simulink model "loberotator_final"  (R2018a)
settings: Solver=VariableStepAuto  StartTime=0.0  StopTime=100  RelTol=1e-3
libraries: xbsIndex_r4 x104, xps_library x4, casper_library_misc x1
(part 3 of 4)

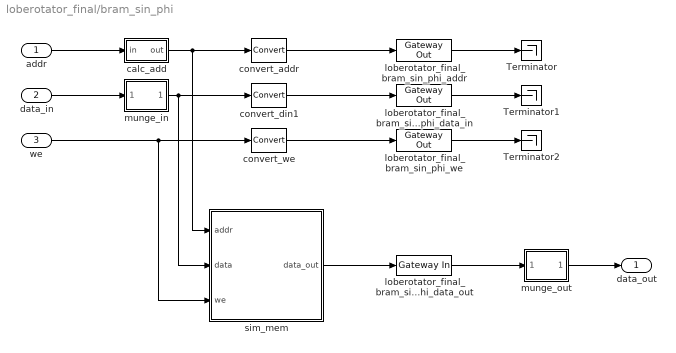
== system loberotator_final/bram_sin_phi ==
  addr : Inport
  data_in : Inport  Port=2
  we : Inport  Port=3
  Terminator : Terminator
  Terminator1 : Terminator
  Terminator2 : Terminator
  calc_add : Subsystem  mask{data_width=32, addr_width=11, sample_rate=sample_rate}
      mask prompts: data_width "data width"; addr_width "address width"; sample_rate "sample rate"
  convert_addr : xbsIndex_r4/Convert  gui_display_data_type=Fixed-point  arith_type=Unsigned  n_bits=addr_width  bin_pt=0  float_type=Single  exp_bits=8  fraction_bits=24  quantization=Truncate  overflow=Wrap  en=off  latency=0  pipeline=off  dbl_ovrd=off  block_type=convert
      settings: xl_area=[0, 0, 0, 0, 0, 0, 0]
  convert_din1 : xbsIndex_r4/Convert  gui_display_data_type=Fixed-point  arith_type=Unsigned  n_bits=32  bin_pt=0  float_type=Single  exp_bits=8  fraction_bits=24  quantization=Truncate  overflow=Wrap  en=off  latency=0  pipeline=off  dbl_ovrd=off  block_type=convert
      settings: xl_area=[0, 0, 0, 0, 0, 0, 0]
  convert_we : xbsIndex_r4/Convert  gui_display_data_type=Fixed-point  arith_type=Unsigned  n_bits=1  bin_pt=0  float_type=Single  exp_bits=8  fraction_bits=24  quantization=Truncate  overflow=Wrap  en=off  latency=0  pipeline=off  dbl_ovrd=off  block_type=convert
      settings: xl_area=[0, 0, 0, 0, 0, 0, 0]
  loberotator_final_bram_sin_phi_addr : xbsIndex_r4/Gateway Out  inherit_from_input=off  hdl_port=on  rows=1  columns=1  UseAsDAC=off  DACChannel='1'  interface=None  automatic_assignment=on  address_offset=hex2dec('00')  intf_name=''  intf_description=''  timing_constraint=None  locs_specified=off  LOCs={'A5','B9','A9','C1','A3','G6','E9','A6','A7','A8','B8','B1','B3','D9','B5','B4','B6','C2'}  io_standard={}  block_type=gatewayout
      settings: infoedit="Gateway out block.  Converts Xilinx fixed point inputs into ouputs of type Simulink integer, double, or fixed point.<P><P>Hardware notes:  In hardware these blocks become top level output ports or are discarded, depending on how they are configured."  sginterface={'Nallatech'=>{'xdspkit'=>{'non_memory_mapped_port'=>'uprev_Shared_BRAM_addr'}},'Xilinx'=>{'jtaghwcosim'=>{'non_memory_mapped_port'=>'uprev_Shared_BRAM_addr'},'xdspkit'=>{'non_memory_mapped_port'=>'uprev_Shared_BRAM_addr'}}}  xl_area=[0, 0, 0, 0, 0, 0, 0]
  loberotator_final_bram_sin_phi_data_in : xbsIndex_r4/Gateway Out  inherit_from_input=off  hdl_port=on  rows=1  columns=1  UseAsDAC=off  DACChannel='1'  interface=None  automatic_assignment=on  address_offset=hex2dec('00')  intf_name=''  intf_description=''  timing_constraint=None  locs_specified=off  LOCs={'B21','B22','A22','B23','B19','C19','A20','A21','A23','B24','A24','A25','E18','D18','C18','B18'}  io_standard={}  block_type=gatewayout
      settings: infoedit="Gateway out block.  Converts Xilinx fixed point inputs into ouputs of type Simulink integer, double, or fixed point.<P><P>Hardware notes:  In hardware these blocks become top level output ports or are discarded, depending on how they are configured."  sginterface={'Nallatech'=>{'xdspkit'=>{'non_memory_mapped_port'=>'uprev_Shared_BRAM_data_in'}},'Xilinx'=>{'jtaghwcosim'=>{'non_memory_mapped_port'=>'uprev_Shared_BRAM_data_in'},'xdspkit'=>{'non_memory_mapped_port'=>'uprev_Shared_BRAM_data_in'}}}  xl_area=[0, 0, 0, 0, 0, 0, 0]
  loberotator_final_bram_sin_phi_data_out : xbsIndex_r4/Gateway In  gui_display_data_type=Fixed-point  arith_type=Unsigned  n_bits=32  bin_pt=0  preci_type=Single  exp_width=8  frac_width=24  rows=1  columns=1  quantization=Truncate  overflow=Wrap  period=sample_rate  UseAsADC=off  ADCChannel='1'  interface=None  automatic_assignment=on  address_offset=hex2dec('00')  intf_name=''  intf_description=''  default_value=0  timing_constraint=None  locs_specified=off  LOCs={}  io_standard={}  inherit_from_input=off  hdl_port=on  dbl_ovrd=off  block_type=gatewayin
      settings: xl_area=[0, 0, 0, 0, 0, 0, 0]
  loberotator_final_bram_sin_phi_we : xbsIndex_r4/Gateway Out  inherit_from_input=off  hdl_port=on  rows=1  columns=1  UseAsDAC=off  DACChannel='1'  interface=None  automatic_assignment=on  address_offset=hex2dec('00')  intf_name=''  intf_description=''  timing_constraint=None  locs_specified=off  LOCs={'A14'}  io_standard={}  block_type=gatewayout
      settings: infoedit="Gateway out block.  Converts Xilinx fixed point inputs into ouputs of type Simulink integer, double, or fixed point.<P><P>Hardware notes:  In hardware these blocks become top level output ports or are discarded, depending on how they are configured."  xl_area=[0, 0, 0, 0, 0, 0, 0]
  munge_in : Subsystem  AncestorBlock=casper_library_flow_control/munge  mask(munge){divisions=1, div_size=32, order=[0], arith_type_out=Unsigned, bin_pt_out=0}
      mask prompts: divisions "Number of divisions"; div_size "Division size (bits)"; order "Division packing order"; arith_type_out "Output arithmetic type"; bin_pt_out "Output binary point"
      mask help: Splits an input bus into the specified number of divisions and then recombines them in the order specified (most significant division = 0,least = number divisions-1)
      mask init:
      | munge_init(gcb, ...
      |     'divisions', divisions, ...
      |     'div_size', div_size, ...
      |     'order', order, ...
      |     'arith_type_out', arith_type_out, ...
      |     'bin_pt_out', bin_pt_out);
      settings: AttributesFormatString=|
      | split:32
      | join:0
      | Unsigned [32,0]
      mask TypeOptions arith_type_out: Unsigned | Signed  (2's comp) | Floating-point
  munge_out : Subsystem  AncestorBlock=casper_library_flow_control/munge  mask(munge){divisions=1, div_size=32, order=[0], arith_type_out=Signed  (2's comp), bin_pt_out=0}
      mask prompts: divisions "Number of divisions"; div_size "Division size (bits)"; order "Division packing order"; arith_type_out "Output arithmetic type"; bin_pt_out "Output binary point"
      mask help: Splits an input bus into the specified number of divisions and then recombines them in the order specified (most significant division = 0,least = number divisions-1)
      mask init:
      | munge_init(gcb, ...
      |     'divisions', divisions, ...
      |     'div_size', div_size, ...
      |     'order', order, ...
      |     'arith_type_out', arith_type_out, ...
      |     'bin_pt_out', bin_pt_out);
      settings: AttributesFormatString=|
      | split:32
      | join:0
      | Signed  (2's comp) [32,0]
      mask TypeOptions arith_type_out: Unsigned | Signed  (2's comp) | Floating-point
  sim_mem : Subsystem  mask{arith_type=Signed  (2's comp), addr_width=11, data_width=32, data_bin_pt=0, init_vals=[0      6591605.5285268      13183148.953719      19774568.172827      26365801.084272       32956785.58823      39547459.587217      46137760.986676      52727627.695558      59316997.626911      65905808.698464       72493998.83321      79081505.959994      85668268.014094      92254222.937808       98839308.68104      105423463.20188       112006624.4672      118588730.45322       125169719.1461      131749528.54254      138328096.65034        144905361.489       151481261.0903      158055733.49888      164628716.77283      171200148.98425      177769968.21988      184338112.58165      190904520.18727       197469129.1708      204031877.68326      210592703.89319      217151545.98725      223708342.17079      230263030.66843      236815549.72465      243365837.60438      249913832.59356      256459472.99973      263002697.15263      269543443.40474      276081650.13191      282617255.73391        289150198.635      295680417.28456       302207850.1576      308732435.75539      315254112.60604      321772819.26506      328288494.31592      334801076.37068      341310504.07054      347816716.08639      354319651.11945       360819247.9018      367315445.19698      373808181.80054      380297396.54065      386783028.27866      393265015.90968      399743298.36314       406217814.6034      412688503.63028      419155304.47967       425618156.2241      432076997.97329      438531768.87477      444982408.11438      451428854.91692      457871048.54668      464308928.30802      470742433.54595      477171503.64669      483596078.03824      490016096.19096      496431497.61815      502842221.87659      509248208.56713      515649397.33527      522045727.87168      528437139.91285      534823573.24157      541204967.68755      547581263.12798      553952399.48808       560318316.7417      566678954.91183      573034254.07122      579384154.34291      585728595.90081      592067518.97027      598400863.82861      604728570.80572      611050580.28462      617366832.70199      623677268.54875      629981828.37063      636280452.76873      642573082.40004      648859657.97807      655140120.27334      661414410.11398      667682468.38627       673944236.0352      680199654.06503      686448663.53983      692691205.58409      698927221.38318      705156652.18399      711379439.29544      717595524.08905      723804847.99949      730007352.52512      736202979.22854      742391669.73718      748573365.74378      754748009.00702        760915541.352      767075904.67082      773229040.92313      779374892.13667      785513400.40783      791644507.90214       797768156.8549      803884289.57167       809992848.4288      816093775.87404      822187014.42701      828272506.67978       834350195.2974      840420023.01844      846481932.65555      852535867.09595      858581769.30203      864619582.31183      870649249.23963      876670713.27644      882683917.69055      888688805.82809      894685321.11352       900673407.0502       906653007.2209      912624065.28835      918586524.99574       924540330.1673      930485424.70877      936421752.60796      942349257.93531      948267884.84434      954177577.57225      960078280.44039      965969937.85482      971852494.30683      977725894.37344      983590082.71795      989445004.09045      995290603.32832      1001126825.3568      1006953615.1894      1012770917.9287      1018578678.7663      1024376842.9842      1030165355.9543      1035944163.1397       1041713210.095      1047472442.4667      1053221805.9936      1058961246.5077      1064690709.9343       1070410142.293      1076119489.6975      1081818698.3569      1087507714.5756       1093186484.754      1098854955.3892      1104513073.0753      1110160784.5038      1115798036.4643      1121424775.8452      1127040949.6335       1132646504.916      1138241388.8796      1143825548.8117      1149398932.1006      1154961486.2362      1160513158.8106      1166053897.5181      1171583650.1563      1177102364.6261      1182609988.9326 ...(+38992 chars)], sample_rate=1, csp_latency=1}
      mask prompts: arith_type "Output Data Type"; addr_width "Address width"; data_width "Data width"; data_bin_pt "Data Binary Point"; init_vals "Initial values"; sample_rate "Sample rate"; csp_latency "Latency"
      mask init:
      | % set_param([gcb, '/data_to_xilinx'], 'arith_type', arith_type)
      | % set_param([gcb, '/data_to_xilinx'], 'n_bits', get_param(gcb, 'data_width'))
      mask TypeOptions arith_type: Unsigned | Signed  (2's comp)
      mask TypeOptions data_width: 8 | 16 | 32 | 64 | 128
  data_out : Outport
  wires:
  munge_out/1(dout) -> data_out/1
  sim_mem/1(data_out) -> loberotator_final_bram_sin_phi_data_out/1
  loberotator_final_bram_sin_phi_data_out/1 -> munge_out/1(din)
  convert_addr/1 -> loberotator_final_bram_sin_phi_addr/1
  convert_din1/1 -> loberotator_final_bram_sin_phi_data_in/1
  data_in/1 -> munge_in/1(din)
  calc_add/1(out) -> sim_mem/1(addr), convert_addr/1
  loberotator_final_bram_sin_phi_we/1 -> Terminator2/1
  loberotator_final_bram_sin_phi_data_in/1 -> Terminator1/1
  loberotator_final_bram_sin_phi_addr/1 -> Terminator/1
  convert_we/1 -> loberotator_final_bram_sin_phi_we/1
  addr/1 -> calc_add/1(in)
  we/1 -> sim_mem/3(we), convert_we/1
  munge_in/1(dout) -> sim_mem/2(data), convert_din1/1
